simulink model "test_p53_compare_with_chip_20160118"  (R2014a)
settings: Solver=ode15s  StartTime=0.0  StopTime=0.452  FixedStep=0.001e-3  RelTol=1e-8  AbsTol=1e-11
values from neighbouring files (symbols this model uses):
  KDfw = 10    [test_p53_compare_with_chip_20160118_Sim.m]
  KDfw_b2 = 0.724    [test_p53_compare_with_chip_20160118_Sim.m]
  KDfw_b8 = 0.5    [test_p53_compare_with_chip_20160118_Sim.m]
  KDrv = 10    [test_p53_compare_with_chip_20160118_Sim.m]
  kr1_b1 = 197.24    [test_p53_compare_with_chip_20160118_Sim.m]
  kr1_b2 = 200    [test_p53_compare_with_chip_20160118_Sim.m]
  kr1_b3 = 23.91    [test_p53_compare_with_chip_20160118_Sim.m]
  kr1_b4 = 118.3    [test_p53_compare_with_chip_20160118_Sim.m]
  kr1_b6 = 478    [test_p53_compare_with_chip_20160118_Sim.m]
  kr1_b7 = 7.89    [test_p53_compare_with_chip_20160118_Sim.m]
  kr1_b8 = 1195    [test_p53_compare_with_chip_20160118_Sim.m]
  kr2 = 10    [test_p53_compare_with_chip_20160118_Sim.m]
  kr2_b1 = 197.24    [test_p53_compare_with_chip_20160118_Sim.m]
  kr2_b3 = 23.91    [test_p53_compare_with_chip_20160118_Sim.m]
  kr2_b4 = 239.1    [test_p53_compare_with_chip_20160118_Sim.m]
  kr2_b6 = 4.78    [test_p53_compare_with_chip_20160118_Sim.m]
  kr2_b7 = 23.91    [test_p53_compare_with_chip_20160118_Sim.m]
  kr2_b8 = 239.1    [test_p53_compare_with_chip_20160118_Sim.m]
  n = 1    [test_p53_compare_with_chip_20160118_Sim.m]
  ratC = 0    [test_p53_compare_with_chip_20160118_Sim.m]
  ratC1 = 1    [test_p53_compare_with_chip_20160118_Sim.m]
  ratC_b4 = 0.433    [test_p53_compare_with_chip_20160118_Sim.m]
settings Model: Creator=lorenzo  LastModifiedBy=Sung
settings SolverCC: ZeroCrossControl=DisableAll
settings DataIOCC: SignalLoggingSaveFormat=ModelDataLogs
settings OptimizationCC: ExpressionDepthLimit=2147483647
settings DebuggingCC: UnderspecifiedInitializationDetection=Classic  FcnCallInpInsideContextMsg=UseLocalSettings  StateNameClashWarn=warning
settings GRTTargetCC: CombineOutputUpdateFcns=off  GRTInterface=on

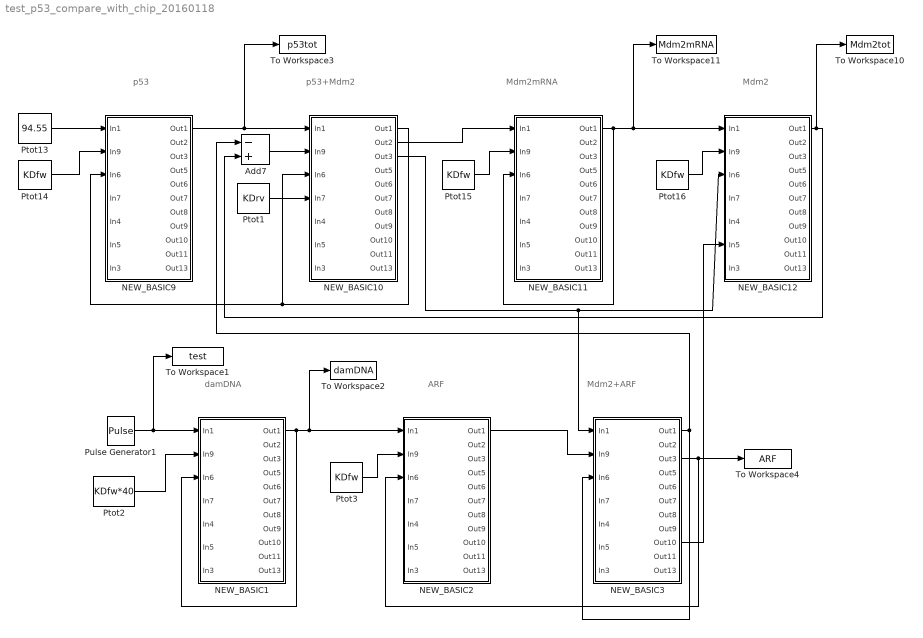
== system test_p53_compare_with_chip_20160118 ==
  note: p53
  note: p53+Mdm2
  note: Mdm2mRNA
  note: Mdm2
  note: damDNA
  note: ARF
  note: Mdm2+ARF
  Add7 : Sum  Inputs=-+
  NEW_BASIC1 : Subsystem
  NEW_BASIC10 : Subsystem
  NEW_BASIC11 : Subsystem
  NEW_BASIC12 : Subsystem
  NEW_BASIC2 : Subsystem
  NEW_BASIC3 : Subsystem
  NEW_BASIC9 : Subsystem
  Ptot1 : Constant  Value=KDrv
  Ptot13 : Constant  Value=94.55
  Ptot{3,14..16} (4 alike) : Constant  Value=KDfw
  Ptot2 : Constant  Value=KDfw*40
  Pulse Generator1 : DiscretePulseGenerator  PulseType=Time based  Amplitude=25  Period=100  PulseWidth=0.000251  PhaseDelay=0.015
  To Workspace1 : ToWorkspace  VariableName=test  SaveFormat=Timeseries  SampleTime=-1
  To Workspace10 : ToWorkspace  VariableName=Mdm2tot  SaveFormat=Timeseries  SampleTime=-1
  To Workspace11 : ToWorkspace  VariableName=Mdm2mRNA  SaveFormat=Timeseries  SampleTime=-1
  To Workspace2 : ToWorkspace  VariableName=damDNA  SaveFormat=Timeseries  SampleTime=-1
  To Workspace3 : ToWorkspace  VariableName=p53tot  SaveFormat=Timeseries  SampleTime=-1
  To Workspace4 : ToWorkspace  VariableName=ARF  SaveFormat=Timeseries  SampleTime=-1
  wires:
  Ptot13/1 -> NEW_BASIC9/1(In1)
  Ptot14/1 -> NEW_BASIC9/2(In9)
  NEW_BASIC9/1(Out1) -> To Workspace3/1, NEW_BASIC10/1(In1)
  NEW_BASIC10/1(Out1) -> NEW_BASIC10/3(In6), NEW_BASIC9/3(In6)
  NEW_BASIC11/1(Out1) -> To Workspace11/1, NEW_BASIC12/1(In1), NEW_BASIC11/3(In6)
  NEW_BASIC10/2(Out2) -> NEW_BASIC11/1(In1)
  Ptot15/1 -> NEW_BASIC11/2(In9)
  Ptot16/1 -> NEW_BASIC12/2(In9)
  NEW_BASIC12/1(Out1) -> Add7/2, To Workspace10/1
  NEW_BASIC10/3(Out3) -> NEW_BASIC12/3(In6), NEW_BASIC3/1(In1)
  Ptot1/1 -> NEW_BASIC10/4(In7)
  Pulse Generator1/1 -> To Workspace1/1, NEW_BASIC1/1(In1)
  Ptot2/1 -> NEW_BASIC1/2(In9)
  NEW_BASIC1/1(Out1) -> To Workspace2/1, NEW_BASIC2/1(In1), NEW_BASIC1/3(In6)
  Ptot3/1 -> NEW_BASIC2/2(In9)
  NEW_BASIC2/1(Out1) -> NEW_BASIC3/2(In9)
  NEW_BASIC3/3(Out3) -> To Workspace4/1, NEW_BASIC2/3(In6)
  NEW_BASIC3/9(Out10) -> NEW_BASIC12/6(In5)
  Add7/1 -> NEW_BASIC10/2(In9)
  NEW_BASIC3/1(Out1) -> Add7/1, NEW_BASIC3/3(In6)

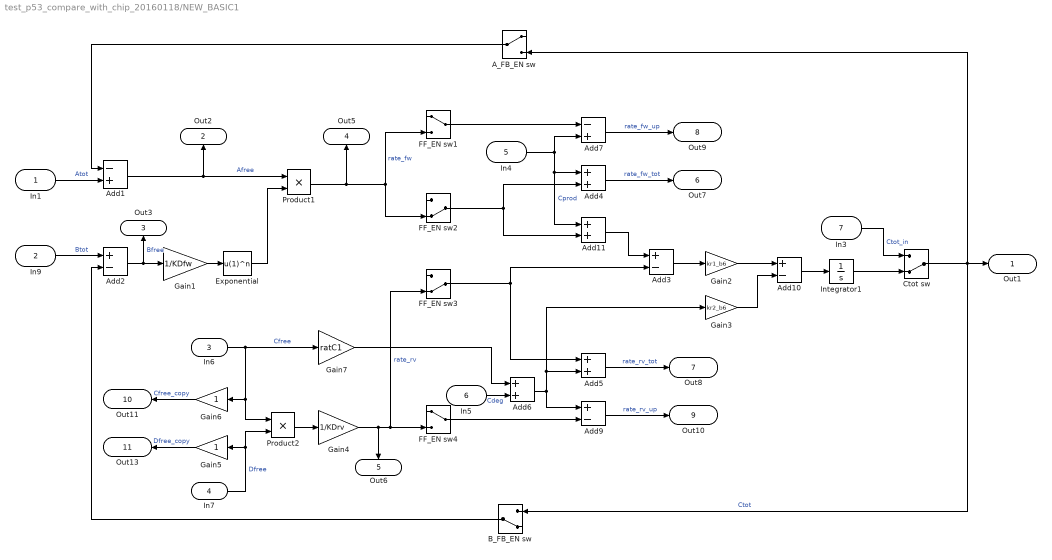
== system test_p53_compare_with_chip_20160118/NEW_BASIC1 ==
  In1 : Inport
  In9 : Inport  Port=2
  In6 : Inport  Port=3
  In7 : Inport  Port=4
  In4 : Inport  Port=5
  In5 : Inport  Port=6
  In3 : Inport  Port=7
  A_FB_EN sw : ManualSwitch
  Add1 : Sum  Inputs=-+
  Add{2..3,9..10} (4 alike) : Sum  Inputs=+-
  Add{4..6,11} (4 alike) : Sum
  Add7 : Sum  Inputs=-+
  B_FB_EN sw : ManualSwitch  CurrentSetting=0
  Ctot sw : ManualSwitch  CurrentSetting=0
  Exponential : Fcn  Expr=u(1)^n
  FF_EN sw1 : ManualSwitch
  FF_EN sw2 : ManualSwitch  CurrentSetting=0
  FF_EN sw3 : ManualSwitch  CurrentSetting=0
  FF_EN sw4 : ManualSwitch
  Gain1 : Gain  Gain=1/KDfw
  Gain2 : Gain  Gain=kr1_b6
  Gain3 : Gain  Gain=kr2_b6
  Gain4 : Gain  Gain=1/KDrv
  Gain5 : Gain
  Gain6 : Gain
  Gain7 : Gain  Gain=ratC1
  Integrator1 : Integrator
  Product1 : Product  RndMeth=Zero
  Product2 : Product  RndMeth=Zero
  Out1 : Outport
  Out2 : Outport  Port=2
  Out3 : Outport  Port=3
  Out5 : Outport  Port=4
  Out6 : Outport  Port=5
  Out7 : Outport  Port=6
  Out8 : Outport  Port=7
  Out9 : Outport  Port=8
  Out10 : Outport  Port=9
  Out11 : Outport  Port=10
  Out13 : Outport  Port=11
  wires:
  FF_EN sw3/1 -> Add5/1, Add3/2
  Add11/1 -> Add3/1
  Gain3/1 -> Add10/2
  Gain2/1 -> Add10/1
  Add10/1 -> Integrator1/1
  Gain7/1 -> Add6/1
  Add5/1 -> Out8/1  "rate_rv_tot"
  Add6/1 -> Add9/1, Add5/2, Gain3/1
  FF_EN sw4/1 -> Add9/2
  Gain4/1 -> FF_EN sw3/2, FF_EN sw4/2, Out6/1  "rate_rv"
  Gain6/1 -> Out11/1  "Cfree_copy"
  Product2/1 -> Gain4/1
  In7/1 -> Gain5/1, Product2/2  "Dfree"
  In6/1 -> Gain7/1, Product2/1, Gain6/1  "Cfree"
  In5/1 -> Add6/2  "Cdeg"
  FF_EN sw1/1 -> Add7/1
  Ctot sw/1 -> B_FB_EN sw/1, A_FB_EN sw/2, Out1/1  "Ctot"
  Integrator1/1 -> Ctot sw/2
  Add9/1 -> Out10/1  "rate_rv_up"
  Add7/1 -> Out9/1  "rate_fw_up"
  Add4/1 -> Out7/1  "rate_fw_tot"
  In4/1 -> Add7/2, Add4/1, Add11/1  "Cprod"
  Product1/1 -> FF_EN sw1/2, FF_EN sw2/2, Out5/1  "rate_fw"
  Exponential/1 -> Product1/2
  Gain1/1 -> Exponential/1
  In9/1 -> Add2/1  "Btot"
  In1/1 -> Add1/2  "Atot"
  Add1/1 -> Product1/1, Out2/1  "Afree"
  Add2/1 -> Out3/1, Gain1/1  "Bfree"
  Add3/1 -> Gain2/1
  A_FB_EN sw/1 -> Add1/1
  B_FB_EN sw/1 -> Add2/2
  Gain5/1 -> Out13/1  "Dfree_copy"
  In3/1 -> Ctot sw/1  "Ctot_in"
  FF_EN sw2/1 -> Add4/2, Add11/2

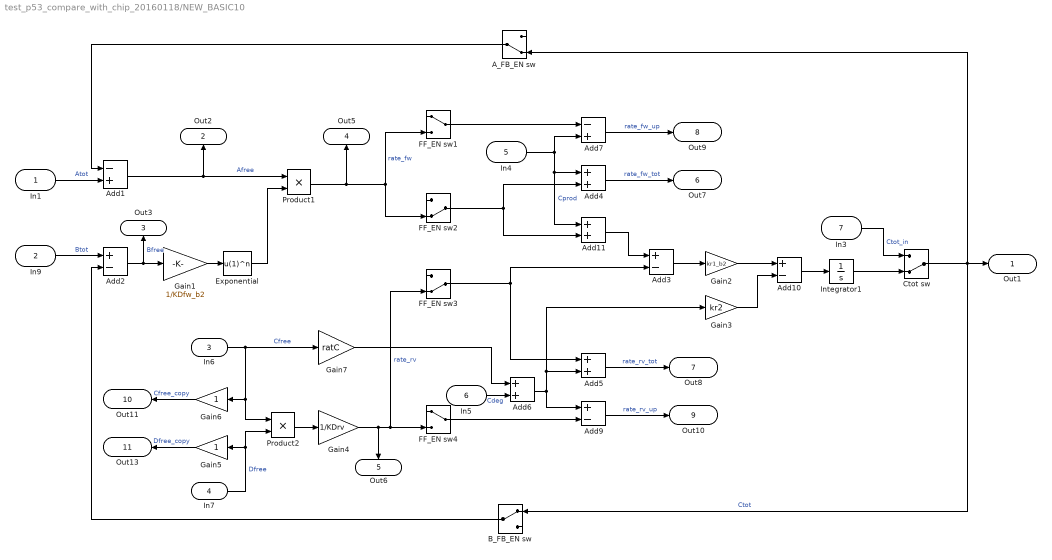
== system test_p53_compare_with_chip_20160118/NEW_BASIC10 ==
  In1 : Inport
  In9 : Inport  Port=2
  In6 : Inport  Port=3
  In7 : Inport  Port=4
  In4 : Inport  Port=5
  In5 : Inport  Port=6
  In3 : Inport  Port=7
  A_FB_EN sw : ManualSwitch  CurrentSetting=0
  Add1 : Sum  Inputs=-+
  Add{2..3,9..10} (4 alike) : Sum  Inputs=+-
  Add{4..6,11} (4 alike) : Sum
  Add7 : Sum  Inputs=-+
  B_FB_EN sw : ManualSwitch
  Ctot sw : ManualSwitch  CurrentSetting=0
  Exponential : Fcn  Expr=u(1)^n
  FF_EN sw1 : ManualSwitch
  FF_EN sw2 : ManualSwitch  CurrentSetting=0
  FF_EN sw3 : ManualSwitch  CurrentSetting=0
  FF_EN sw4 : ManualSwitch
  Gain1 : Gain  Gain=1/KDfw_b2
  Gain2 : Gain  Gain=kr1_b2
  Gain3 : Gain  Gain=kr2
  Gain4 : Gain  Gain=1/KDrv
  Gain5 : Gain
  Gain6 : Gain
  Gain7 : Gain  Gain=ratC
  Integrator1 : Integrator  InitialCondition=95
  Product1 : Product  RndMeth=Zero
  Product2 : Product  RndMeth=Zero
  Out1 : Outport
  Out2 : Outport  Port=2
  Out3 : Outport  Port=3
  Out5 : Outport  Port=4
  Out6 : Outport  Port=5
  Out7 : Outport  Port=6
  Out8 : Outport  Port=7
  Out9 : Outport  Port=8
  Out10 : Outport  Port=9
  Out11 : Outport  Port=10
  Out13 : Outport  Port=11
  wires:
  FF_EN sw3/1 -> Add5/1, Add3/2
  Add11/1 -> Add3/1
  Gain3/1 -> Add10/2
  Gain2/1 -> Add10/1
  Add10/1 -> Integrator1/1
  Gain7/1 -> Add6/1
  Add5/1 -> Out8/1  "rate_rv_tot"
  Add6/1 -> Add9/1, Add5/2, Gain3/1
  FF_EN sw4/1 -> Add9/2
  Gain4/1 -> FF_EN sw3/2, FF_EN sw4/2, Out6/1  "rate_rv"
  Gain6/1 -> Out11/1  "Cfree_copy"
  Product2/1 -> Gain4/1
  In7/1 -> Gain5/1, Product2/2  "Dfree"
  In6/1 -> Gain7/1, Product2/1, Gain6/1  "Cfree"
  In5/1 -> Add6/2  "Cdeg"
  FF_EN sw1/1 -> Add7/1
  Ctot sw/1 -> B_FB_EN sw/1, A_FB_EN sw/2, Out1/1  "Ctot"
  Integrator1/1 -> Ctot sw/2
  Add9/1 -> Out10/1  "rate_rv_up"
  Add7/1 -> Out9/1  "rate_fw_up"
  Add4/1 -> Out7/1  "rate_fw_tot"
  In4/1 -> Add7/2, Add4/1, Add11/1  "Cprod"
  Product1/1 -> FF_EN sw1/2, FF_EN sw2/2, Out5/1  "rate_fw"
  Exponential/1 -> Product1/2
  Gain1/1 -> Exponential/1
  In9/1 -> Add2/1  "Btot"
  In1/1 -> Add1/2  "Atot"
  Add1/1 -> Product1/1, Out2/1  "Afree"
  Add2/1 -> Out3/1, Gain1/1  "Bfree"
  Add3/1 -> Gain2/1
  A_FB_EN sw/1 -> Add1/1
  B_FB_EN sw/1 -> Add2/2
  Gain5/1 -> Out13/1  "Dfree_copy"
  In3/1 -> Ctot sw/1  "Ctot_in"
  FF_EN sw2/1 -> Add4/2, Add11/2

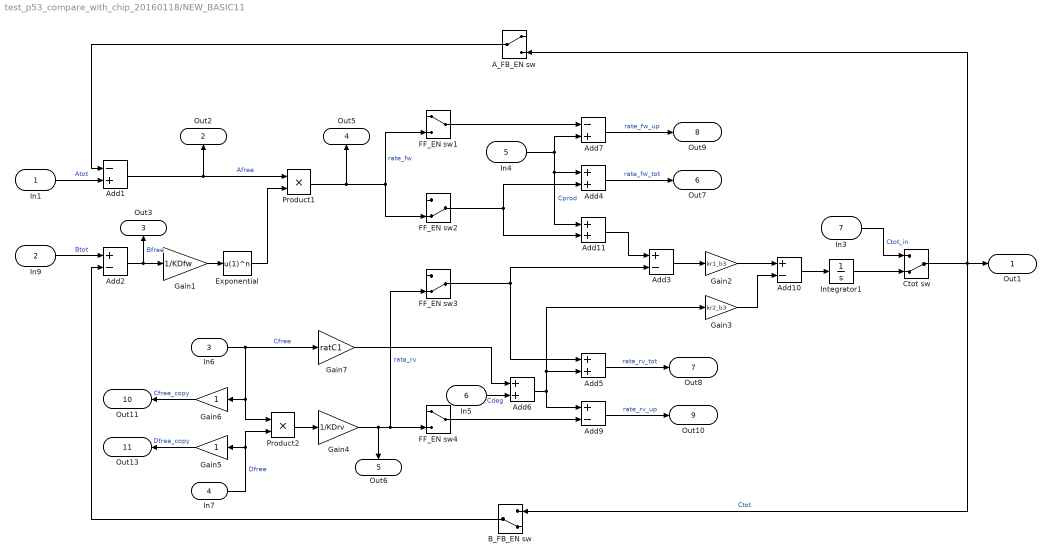
== system test_p53_compare_with_chip_20160118/NEW_BASIC11 ==
  In1 : Inport
  In9 : Inport  Port=2
  In6 : Inport  Port=3
  In7 : Inport  Port=4
  In4 : Inport  Port=5
  In5 : Inport  Port=6
  In3 : Inport  Port=7
  A_FB_EN sw : ManualSwitch
  Add1 : Sum  Inputs=-+
  Add{2..3,9..10} (4 alike) : Sum  Inputs=+-
  Add{4..6,11} (4 alike) : Sum
  Add7 : Sum  Inputs=-+
  B_FB_EN sw : ManualSwitch  CurrentSetting=0
  Ctot sw : ManualSwitch  CurrentSetting=0
  Exponential : Fcn  Expr=u(1)^n
  FF_EN sw1 : ManualSwitch
  FF_EN sw2 : ManualSwitch  CurrentSetting=0
  FF_EN sw3 : ManualSwitch  CurrentSetting=0
  FF_EN sw4 : ManualSwitch
  Gain1 : Gain  Gain=1/KDfw
  Gain2 : Gain  Gain=kr1_b3
  Gain3 : Gain  Gain=kr2_b3
  Gain4 : Gain  Gain=1/KDrv
  Gain5 : Gain
  Gain6 : Gain
  Gain7 : Gain  Gain=ratC1
  Integrator1 : Integrator
  Product1 : Product  RndMeth=Zero
  Product2 : Product  RndMeth=Zero
  Out1 : Outport
  Out2 : Outport  Port=2
  Out3 : Outport  Port=3
  Out5 : Outport  Port=4
  Out6 : Outport  Port=5
  Out7 : Outport  Port=6
  Out8 : Outport  Port=7
  Out9 : Outport  Port=8
  Out10 : Outport  Port=9
  Out11 : Outport  Port=10
  Out13 : Outport  Port=11
  wires:
  FF_EN sw2/1 -> Add11/2, Add4/2
  In3/1 -> Ctot sw/1  "Ctot_in"
  Gain5/1 -> Out13/1  "Dfree_copy"
  B_FB_EN sw/1 -> Add2/2
  A_FB_EN sw/1 -> Add1/1
  Add3/1 -> Gain2/1
  Add2/1 -> Gain1/1, Out3/1  "Bfree"
  Add1/1 -> Out2/1, Product1/1  "Afree"
  In1/1 -> Add1/2  "Atot"
  In9/1 -> Add2/1  "Btot"
  Gain1/1 -> Exponential/1
  Exponential/1 -> Product1/2
  Product1/1 -> Out5/1, FF_EN sw2/2, FF_EN sw1/2  "rate_fw"
  In4/1 -> Add11/1, Add4/1, Add7/2  "Cprod"
  Add4/1 -> Out7/1  "rate_fw_tot"
  Add7/1 -> Out9/1  "rate_fw_up"
  Add9/1 -> Out10/1  "rate_rv_up"
  Integrator1/1 -> Ctot sw/2
  Ctot sw/1 -> Out1/1, A_FB_EN sw/2, B_FB_EN sw/1  "Ctot"
  FF_EN sw1/1 -> Add7/1
  In5/1 -> Add6/2  "Cdeg"
  In6/1 -> Gain6/1, Product2/1, Gain7/1  "Cfree"
  In7/1 -> Product2/2, Gain5/1  "Dfree"
  Product2/1 -> Gain4/1
  Gain6/1 -> Out11/1  "Cfree_copy"
  Gain4/1 -> Out6/1, FF_EN sw4/2, FF_EN sw3/2  "rate_rv"
  FF_EN sw4/1 -> Add9/2
  Add6/1 -> Gain3/1, Add5/2, Add9/1
  Add5/1 -> Out8/1  "rate_rv_tot"
  Gain7/1 -> Add6/1
  Add10/1 -> Integrator1/1
  Gain2/1 -> Add10/1
  Gain3/1 -> Add10/2
  Add11/1 -> Add3/1
  FF_EN sw3/1 -> Add3/2, Add5/1

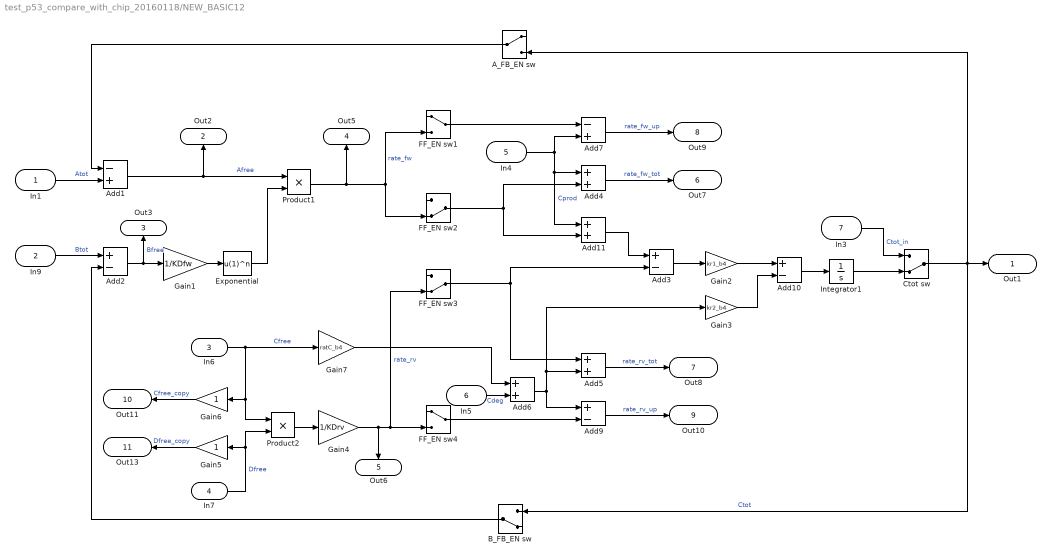
== system test_p53_compare_with_chip_20160118/NEW_BASIC12 ==
  In1 : Inport
  In9 : Inport  Port=2
  In6 : Inport  Port=3
  In7 : Inport  Port=4
  In4 : Inport  Port=5
  In5 : Inport  Port=6
  In3 : Inport  Port=7
  A_FB_EN sw : ManualSwitch
  Add1 : Sum  Inputs=-+
  Add{2..3,9..10} (4 alike) : Sum  Inputs=+-
  Add{4..6,11} (4 alike) : Sum
  Add7 : Sum  Inputs=-+
  B_FB_EN sw : ManualSwitch  CurrentSetting=0
  Ctot sw : ManualSwitch  CurrentSetting=0
  Exponential : Fcn  Expr=u(1)^n
  FF_EN sw1 : ManualSwitch
  FF_EN sw2 : ManualSwitch  CurrentSetting=0
  FF_EN sw3 : ManualSwitch  CurrentSetting=0
  FF_EN sw4 : ManualSwitch
  Gain1 : Gain  Gain=1/KDfw
  Gain2 : Gain  Gain=kr1_b4
  Gain3 : Gain  Gain=kr2_b4
  Gain4 : Gain  Gain=1/KDrv
  Gain5 : Gain
  Gain6 : Gain
  Gain7 : Gain  Gain=ratC_b4
  Integrator1 : Integrator  InitialCondition=100
  Product1 : Product  RndMeth=Zero
  Product2 : Product  RndMeth=Zero
  Out1 : Outport
  Out2 : Outport  Port=2
  Out3 : Outport  Port=3
  Out5 : Outport  Port=4
  Out6 : Outport  Port=5
  Out7 : Outport  Port=6
  Out8 : Outport  Port=7
  Out9 : Outport  Port=8
  Out10 : Outport  Port=9
  Out11 : Outport  Port=10
  Out13 : Outport  Port=11
  wires:
  FF_EN sw3/1 -> Add5/1, Add3/2
  Add11/1 -> Add3/1
  Gain3/1 -> Add10/2
  Gain2/1 -> Add10/1
  Add10/1 -> Integrator1/1
  Gain7/1 -> Add6/1
  Add5/1 -> Out8/1  "rate_rv_tot"
  Add6/1 -> Add9/1, Add5/2, Gain3/1
  FF_EN sw4/1 -> Add9/2
  Gain4/1 -> FF_EN sw3/2, FF_EN sw4/2, Out6/1  "rate_rv"
  Gain6/1 -> Out11/1  "Cfree_copy"
  Product2/1 -> Gain4/1
  In7/1 -> Gain5/1, Product2/2  "Dfree"
  In6/1 -> Gain7/1, Product2/1, Gain6/1  "Cfree"
  In5/1 -> Add6/2  "Cdeg"
  FF_EN sw1/1 -> Add7/1
  Ctot sw/1 -> B_FB_EN sw/1, A_FB_EN sw/2, Out1/1  "Ctot"
  Integrator1/1 -> Ctot sw/2
  Add9/1 -> Out10/1  "rate_rv_up"
  Add7/1 -> Out9/1  "rate_fw_up"
  Add4/1 -> Out7/1  "rate_fw_tot"
  In4/1 -> Add7/2, Add4/1, Add11/1  "Cprod"
  Product1/1 -> FF_EN sw1/2, FF_EN sw2/2, Out5/1  "rate_fw"
  Exponential/1 -> Product1/2
  Gain1/1 -> Exponential/1
  In9/1 -> Add2/1  "Btot"
  In1/1 -> Add1/2  "Atot"
  Add1/1 -> Product1/1, Out2/1  "Afree"
  Add2/1 -> Out3/1, Gain1/1  "Bfree"
  Add3/1 -> Gain2/1
  A_FB_EN sw/1 -> Add1/1
  B_FB_EN sw/1 -> Add2/2
  Gain5/1 -> Out13/1  "Dfree_copy"
  In3/1 -> Ctot sw/1  "Ctot_in"
  FF_EN sw2/1 -> Add4/2, Add11/2

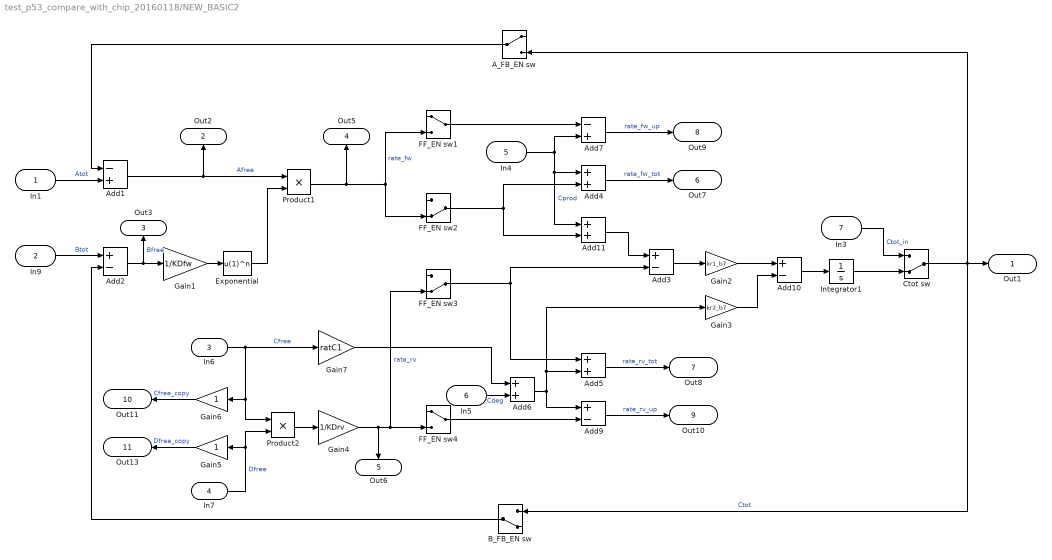
== system test_p53_compare_with_chip_20160118/NEW_BASIC2 ==
  In1 : Inport
  In9 : Inport  Port=2
  In6 : Inport  Port=3
  In7 : Inport  Port=4
  In4 : Inport  Port=5
  In5 : Inport  Port=6
  In3 : Inport  Port=7
  A_FB_EN sw : ManualSwitch
  Add1 : Sum  Inputs=-+
  Add{2..3,9..10} (4 alike) : Sum  Inputs=+-
  Add{4..6,11} (4 alike) : Sum
  Add7 : Sum  Inputs=-+
  B_FB_EN sw : ManualSwitch  CurrentSetting=0
  Ctot sw : ManualSwitch  CurrentSetting=0
  Exponential : Fcn  Expr=u(1)^n
  FF_EN sw1 : ManualSwitch
  FF_EN sw2 : ManualSwitch  CurrentSetting=0
  FF_EN sw3 : ManualSwitch  CurrentSetting=0
  FF_EN sw4 : ManualSwitch
  Gain1 : Gain  Gain=1/KDfw
  Gain2 : Gain  Gain=kr1_b7
  Gain3 : Gain  Gain=kr2_b7
  Gain4 : Gain  Gain=1/KDrv
  Gain5 : Gain
  Gain6 : Gain
  Gain7 : Gain  Gain=ratC1
  Integrator1 : Integrator
  Product1 : Product  RndMeth=Zero
  Product2 : Product  RndMeth=Zero
  Out1 : Outport
  Out2 : Outport  Port=2
  Out3 : Outport  Port=3
  Out5 : Outport  Port=4
  Out6 : Outport  Port=5
  Out7 : Outport  Port=6
  Out8 : Outport  Port=7
  Out9 : Outport  Port=8
  Out10 : Outport  Port=9
  Out11 : Outport  Port=10
  Out13 : Outport  Port=11
  wires:
  FF_EN sw3/1 -> Add5/1, Add3/2
  Add11/1 -> Add3/1
  Gain3/1 -> Add10/2
  Gain2/1 -> Add10/1
  Add10/1 -> Integrator1/1
  Gain7/1 -> Add6/1
  Add5/1 -> Out8/1  "rate_rv_tot"
  Add6/1 -> Add9/1, Add5/2, Gain3/1
  FF_EN sw4/1 -> Add9/2
  Gain4/1 -> FF_EN sw3/2, FF_EN sw4/2, Out6/1  "rate_rv"
  Gain6/1 -> Out11/1  "Cfree_copy"
  Product2/1 -> Gain4/1
  In7/1 -> Gain5/1, Product2/2  "Dfree"
  In6/1 -> Gain7/1, Product2/1, Gain6/1  "Cfree"
  In5/1 -> Add6/2  "Cdeg"
  FF_EN sw1/1 -> Add7/1
  Ctot sw/1 -> B_FB_EN sw/1, A_FB_EN sw/2, Out1/1  "Ctot"
  Integrator1/1 -> Ctot sw/2
  Add9/1 -> Out10/1  "rate_rv_up"
  Add7/1 -> Out9/1  "rate_fw_up"
  Add4/1 -> Out7/1  "rate_fw_tot"
  In4/1 -> Add7/2, Add4/1, Add11/1  "Cprod"
  Product1/1 -> FF_EN sw1/2, FF_EN sw2/2, Out5/1  "rate_fw"
  Exponential/1 -> Product1/2
  Gain1/1 -> Exponential/1
  In9/1 -> Add2/1  "Btot"
  In1/1 -> Add1/2  "Atot"
  Add1/1 -> Product1/1, Out2/1  "Afree"
  Add2/1 -> Out3/1, Gain1/1  "Bfree"
  Add3/1 -> Gain2/1
  A_FB_EN sw/1 -> Add1/1
  B_FB_EN sw/1 -> Add2/2
  Gain5/1 -> Out13/1  "Dfree_copy"
  In3/1 -> Ctot sw/1  "Ctot_in"
  FF_EN sw2/1 -> Add4/2, Add11/2

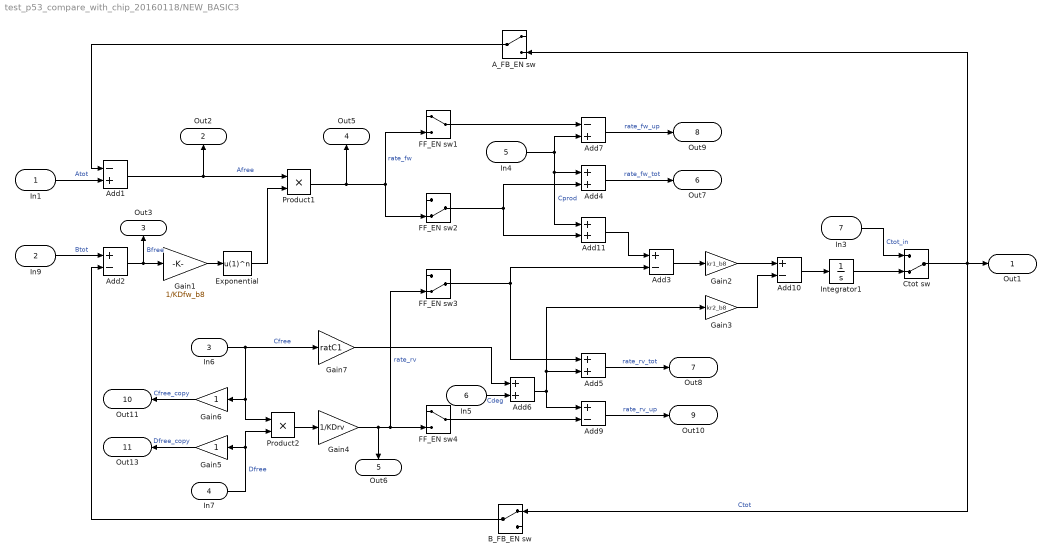
== system test_p53_compare_with_chip_20160118/NEW_BASIC3 ==
  In1 : Inport
  In9 : Inport  Port=2
  In6 : Inport  Port=3
  In7 : Inport  Port=4
  In4 : Inport  Port=5
  In5 : Inport  Port=6
  In3 : Inport  Port=7
  A_FB_EN sw : ManualSwitch
  Add1 : Sum  Inputs=-+
  Add{2..3,9..10} (4 alike) : Sum  Inputs=+-
  Add{4..6,11} (4 alike) : Sum
  Add7 : Sum  Inputs=-+
  B_FB_EN sw : ManualSwitch
  Ctot sw : ManualSwitch  CurrentSetting=0
  Exponential : Fcn  Expr=u(1)^n
  FF_EN sw1 : ManualSwitch
  FF_EN sw2 : ManualSwitch  CurrentSetting=0
  FF_EN sw3 : ManualSwitch  CurrentSetting=0
  FF_EN sw4 : ManualSwitch
  Gain1 : Gain  Gain=1/KDfw_b8
  Gain2 : Gain  Gain=kr1_b8
  Gain3 : Gain  Gain=kr2_b8
  Gain4 : Gain  Gain=1/KDrv
  Gain5 : Gain
  Gain6 : Gain
  Gain7 : Gain  Gain=ratC1
  Integrator1 : Integrator
  Product1 : Product  RndMeth=Zero
  Product2 : Product  RndMeth=Zero
  Out1 : Outport
  Out2 : Outport  Port=2
  Out3 : Outport  Port=3
  Out5 : Outport  Port=4
  Out6 : Outport  Port=5
  Out7 : Outport  Port=6
  Out8 : Outport  Port=7
  Out9 : Outport  Port=8
  Out10 : Outport  Port=9
  Out11 : Outport  Port=10
  Out13 : Outport  Port=11
  wires:
  FF_EN sw2/1 -> Add11/2, Add4/2
  In3/1 -> Ctot sw/1  "Ctot_in"
  Gain5/1 -> Out13/1  "Dfree_copy"
  B_FB_EN sw/1 -> Add2/2
  A_FB_EN sw/1 -> Add1/1
  Add3/1 -> Gain2/1
  Add2/1 -> Gain1/1, Out3/1  "Bfree"
  Add1/1 -> Out2/1, Product1/1  "Afree"
  In1/1 -> Add1/2  "Atot"
  In9/1 -> Add2/1  "Btot"
  Gain1/1 -> Exponential/1
  Exponential/1 -> Product1/2
  Product1/1 -> Out5/1, FF_EN sw2/2, FF_EN sw1/2  "rate_fw"
  In4/1 -> Add11/1, Add4/1, Add7/2  "Cprod"
  Add4/1 -> Out7/1  "rate_fw_tot"
  Add7/1 -> Out9/1  "rate_fw_up"
  Add9/1 -> Out10/1  "rate_rv_up"
  Integrator1/1 -> Ctot sw/2
  Ctot sw/1 -> Out1/1, A_FB_EN sw/2, B_FB_EN sw/1  "Ctot"
  FF_EN sw1/1 -> Add7/1
  In5/1 -> Add6/2  "Cdeg"
  In6/1 -> Gain6/1, Product2/1, Gain7/1  "Cfree"
  In7/1 -> Product2/2, Gain5/1  "Dfree"
  Product2/1 -> Gain4/1
  Gain6/1 -> Out11/1  "Cfree_copy"
  Gain4/1 -> Out6/1, FF_EN sw4/2, FF_EN sw3/2  "rate_rv"
  FF_EN sw4/1 -> Add9/2
  Add6/1 -> Gain3/1, Add5/2, Add9/1
  Add5/1 -> Out8/1  "rate_rv_tot"
  Gain7/1 -> Add6/1
  Add10/1 -> Integrator1/1
  Gain2/1 -> Add10/1
  Gain3/1 -> Add10/2
  Add11/1 -> Add3/1
  FF_EN sw3/1 -> Add3/2, Add5/1

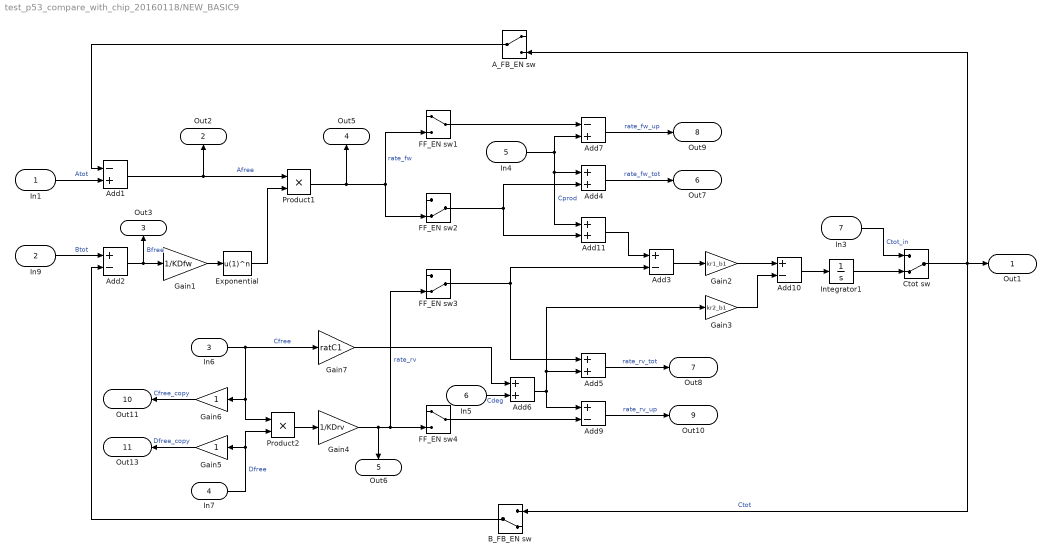
== system test_p53_compare_with_chip_20160118/NEW_BASIC9 ==
  In1 : Inport
  In9 : Inport  Port=2
  In6 : Inport  Port=3
  In7 : Inport  Port=4
  In4 : Inport  Port=5
  In5 : Inport  Port=6
  In3 : Inport  Port=7
  A_FB_EN sw : ManualSwitch
  Add1 : Sum  Inputs=-+
  Add{2..3,9..10} (4 alike) : Sum  Inputs=+-
  Add{4..6,11} (4 alike) : Sum
  Add7 : Sum  Inputs=-+
  B_FB_EN sw : ManualSwitch  CurrentSetting=0
  Ctot sw : ManualSwitch  CurrentSetting=0
  Exponential : Fcn  Expr=u(1)^n
  FF_EN sw1 : ManualSwitch
  FF_EN sw2 : ManualSwitch  CurrentSetting=0
  FF_EN sw3 : ManualSwitch  CurrentSetting=0
  FF_EN sw4 : ManualSwitch
  Gain1 : Gain  Gain=1/KDfw
  Gain2 : Gain  Gain=kr1_b1
  Gain3 : Gain  Gain=kr2_b1
  Gain4 : Gain  Gain=1/KDrv
  Gain5 : Gain
  Gain6 : Gain
  Gain7 : Gain  Gain=ratC1
  Integrator1 : Integrator  InitialCondition=100
  Product1 : Product  RndMeth=Zero
  Product2 : Product  RndMeth=Zero
  Out1 : Outport
  Out2 : Outport  Port=2
  Out3 : Outport  Port=3
  Out5 : Outport  Port=4
  Out6 : Outport  Port=5
  Out7 : Outport  Port=6
  Out8 : Outport  Port=7
  Out9 : Outport  Port=8
  Out10 : Outport  Port=9
  Out11 : Outport  Port=10
  Out13 : Outport  Port=11
  wires:
  FF_EN sw2/1 -> Add11/2, Add4/2
  In3/1 -> Ctot sw/1  "Ctot_in"
  Gain5/1 -> Out13/1  "Dfree_copy"
  B_FB_EN sw/1 -> Add2/2
  A_FB_EN sw/1 -> Add1/1
  Add3/1 -> Gain2/1
  Add2/1 -> Gain1/1, Out3/1  "Bfree"
  Add1/1 -> Out2/1, Product1/1  "Afree"
  In1/1 -> Add1/2  "Atot"
  In9/1 -> Add2/1  "Btot"
  Gain1/1 -> Exponential/1
  Exponential/1 -> Product1/2
  Product1/1 -> Out5/1, FF_EN sw2/2, FF_EN sw1/2  "rate_fw"
  In4/1 -> Add11/1, Add4/1, Add7/2  "Cprod"
  Add4/1 -> Out7/1  "rate_fw_tot"
  Add7/1 -> Out9/1  "rate_fw_up"
  Add9/1 -> Out10/1  "rate_rv_up"
  Integrator1/1 -> Ctot sw/2
  Ctot sw/1 -> Out1/1, A_FB_EN sw/2, B_FB_EN sw/1  "Ctot"
  FF_EN sw1/1 -> Add7/1
  In5/1 -> Add6/2  "Cdeg"
  In6/1 -> Gain6/1, Product2/1, Gain7/1  "Cfree"
  In7/1 -> Product2/2, Gain5/1  "Dfree"
  Product2/1 -> Gain4/1
  Gain6/1 -> Out11/1  "Cfree_copy"
  Gain4/1 -> Out6/1, FF_EN sw4/2, FF_EN sw3/2  "rate_rv"
  FF_EN sw4/1 -> Add9/2
  Add6/1 -> Gain3/1, Add5/2, Add9/1
  Add5/1 -> Out8/1  "rate_rv_tot"
  Gain7/1 -> Add6/1
  Add10/1 -> Integrator1/1
  Gain2/1 -> Add10/1
  Gain3/1 -> Add10/2
  Add11/1 -> Add3/1
  FF_EN sw3/1 -> Add3/2, Add5/1
